simulink model "Pendulum_Plant"  (R2015a)
settings: Solver=ode45  StartTime=0.0  StopTime=10.0  RelTol=1e-3
InitFcn:
  | m = 15;
  | g = 9.81;
  | L = 1.7;
  | b = 2.0;
  | Ts = 0.02;
settings Model: Creator=Logan  LastModifiedBy=Logan
settings DataIOCC: SaveOutput=off  SaveTime=off

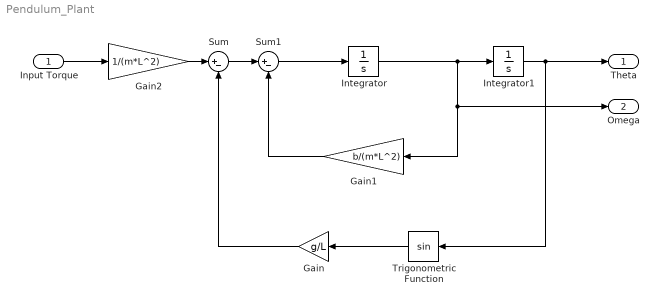
== system Pendulum_Plant ==
  Input Torque : Inport  OutDataTypeStr=double  PortDimensions=1  SampleTime=[0.01,0]
  Gain : Gain  Gain=g/L
  Gain1 : Gain  Gain=b/(m*L^2)
  Gain2 : Gain  Gain=1/(m*L^2)
  Integrator : Integrator
  Integrator1 : Integrator
  Sum : Sum  Inputs=|+-
  Sum1 : Sum  Inputs=|+-
  Trigonometric Function : Trigonometry
  Theta : Outport  OutDataTypeStr=double  PortDimensions=1  SampleTime=0
  Omega : Outport  Port=2  OutDataTypeStr=double  PortDimensions=1  SampleTime=0
  wires:
  Gain/1 -> Sum/2
  Gain1/1 -> Sum1/2
  Sum/1 -> Sum1/1
  Sum1/1 -> Integrator/1
  Input Torque/1 -> Gain2/1
  Gain2/1 -> Sum/1
  Integrator/1 -> Omega/1, Gain1/1, Integrator1/1
  Integrator1/1 -> Trigonometric Function/1, Theta/1
  Trigonometric Function/1 -> Gain/1
